simulink model "sim_pogodowa"  (R2023b)
settings: Solver=VariableStepAuto  StartTime=0.0  StopTime=10.0  FixedStep=0.1  MaxStep=10  RelTol=1e-3
model workspace (MAT data in the model file):
  Var = 0
undefined symbols (not defined in the file): ao, az, bo, bz, cpw, Cvo1, Cvo2, delta_qt1, delta_qt2, delta_Twew_SP, delta_Tzew, deltafmg1, deltafmg2, fmg1_0, fmg2_0, fmw_0, Kco, ki, kp, qt1_0, qt2_0, t_fmg1, t_fmg2, T_gp0, t_op_tr, T_oz0, t_qt1, t_qt2, t_Tzew, t_wew_SP, T_wew_SP_0, T_wp0, T_zew, T_zew0, TwzN
settings Model: Creator=tomasz  LastModifiedBy=tomasz

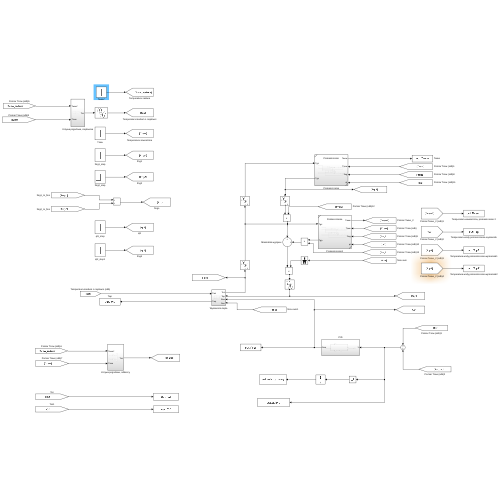
[thumbnail: Simulink's stored preview of the top-level diagram]
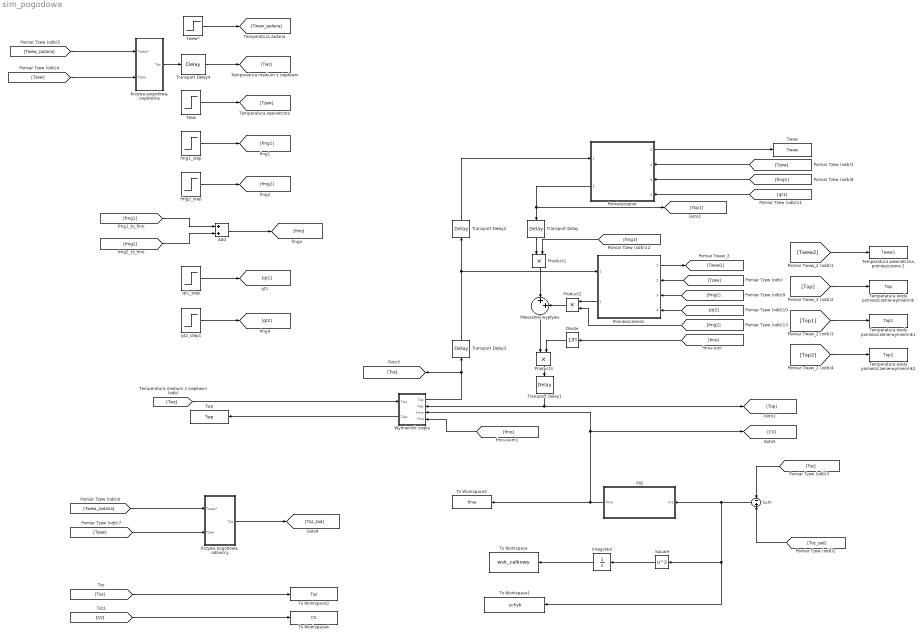
== system sim_pogodowa ==
  Add : Sum
  Divide : Product  Inputs=/
  Integrator : Integrator
  "Krzywa pogodowa, ciepłownia" : Subsystem
  "Krzywa pogodowa, odbiorcy" : Subsystem
  MIeszalnik wypływu : Sum  Inputs=|++
  PID : Subsystem
  Pomieszczenie : Subsystem  ReferencedSubsystem=Pomieszczenie
      settings: PortSchema="{\"entries\":[{\"content\":{\"sides\":[{\"content\":{\"connectorIds\":[\"In1\",\"Out1\"]},\"type\":\"ConnectorPlacement.EquallySpacedRectSide\",\"uuid\":\"8531bf00-72e2-4413-af12-728660d5b7ed\"},{\"content\":{\"connectorIds\":[\"Out2\",\"In2\",\"In3\",\"In4\"],\"side\":\"RIGHT\"},\"type\":\"ConnectorPlacement.EquallySpacedRectSide\",\"uuid\":\"61dc3c29-eecf-49ab-a3f8-5b1de1949346\"},{\"content\":{\"side\":\"TOP\"},\"type\":\"ConnectorPlacement.EquallySpacedRectSide\",\"uuid\":\"a446f5ea-277a-4598-bae9-2c6de6a131a4\"}]},\"type\":\"ConnectorPlacement.EquallySpacedConnector\",\"uuid\":\"c2b24185-542a-4b15-89a0-a367decd74d0\"}],\"packageUris\":[\"http://schema.mathworks.com/mf0/Connector/R2020b\"],\"version\":\"1.0\"}"
  Pomieszczenie1 : Subsystem  ReferencedSubsystem=Pomieszczenie
      settings: PortSchema="{\"entries\":[{\"content\":{\"sides\":[{\"content\":{\"connectorIds\":[\"In1\",\"Out1\"]},\"type\":\"ConnectorPlacement.EquallySpacedRectSide\",\"uuid\":\"8531bf00-72e2-4413-af12-728660d5b7ed\"},{\"content\":{\"connectorIds\":[\"Out2\",\"In2\",\"In3\",\"In4\"],\"side\":\"RIGHT\"},\"type\":\"ConnectorPlacement.EquallySpacedRectSide\",\"uuid\":\"61dc3c29-eecf-49ab-a3f8-5b1de1949346\"},{\"content\":{\"side\":\"TOP\"},\"type\":\"ConnectorPlacement.EquallySpacedRectSide\",\"uuid\":\"a446f5ea-277a-4598-bae9-2c6de6a131a4\"}]},\"type\":\"ConnectorPlacement.EquallySpacedConnector\",\"uuid\":\"c2b24185-542a-4b15-89a0-a367decd74d0\"}],\"packageUris\":[\"http://schema.mathworks.com/mf0/Connector/R2020b\"],\"version\":\"1.0\"}"
  Product1 : Product
  Product2 : Product
  Product3 : Product
  Square : Math  Operator=square
  Sum : Sum  Inputs=-+
  "Temperatura wewnetrzna, pomieszczenie 2" : ToWorkspace  VariableName=Twew1  SampleTime=-1
      settings: Save2DSignal=2-D array (concatenate along first dimension)
  Temperatura wody pomieszczenie-wymiennik : ToWorkspace  VariableName=Top  SampleTime=-1
      settings: Save2DSignal=2-D array (concatenate along first dimension)
  Temperatura wody pomieszczenie-wymiennik1 : ToWorkspace  VariableName=Top1  SaveFormat=Timeseries  SampleTime=-1
  Temperatura wody pomieszczenie-wymiennik2 : ToWorkspace  VariableName=Top2  SaveFormat=Timeseries  SampleTime=-1
  To Workspace : ToWorkspace  VariableName=wsk_calkowy  SampleTime=-1
  To Workspace1 : ToWorkspace  VariableName=uchyb  SampleTime=-1
  To Workspace2 : ToWorkspace  VariableName=fmw  SampleTime=-1
  To Workspace3 : ToWorkspace  VariableName=Toz  SampleTime=-1
  To Workspace4 : ToWorkspace  VariableName=CV  SampleTime=-1
      settings: Save2DSignal=2-D array (concatenate along first dimension)
  Transport Delay : TransportDelay  DelayTime=t_op_tr  InitialOutput=T_gp0
  Transport Delay1 : TransportDelay  DelayTime=t_op_tr  InitialOutput=T_gp0
  Transport Delay2 : TransportDelay  DelayTime=t_op_tr  InitialOutput=T_oz0
  Transport Delay3 : TransportDelay  DelayTime=t_op_tr  InitialOutput=T_oz0
  Transport Delay4 : TransportDelay  DelayTime=1800  InitialOutput=TwzN
  Twew : ToWorkspace  VariableName=Twew  SampleTime=-1
      settings: Save2DSignal=2-D array (concatenate along first dimension)
  Twew* : Step  Time=t_wew_SP  Before=T_wew_SP_0  After=T_wew_SP_0 + delta_Twew_SP  SampleTime=0
  Twp : ToWorkspace  VariableName=Twp  SampleTime=-1
      settings: Save2DSignal=2-D array (concatenate along first dimension)
  Tzew : Step  Time=t_Tzew  Before=T_zew0  After=T_zew + delta_Tzew  SampleTime=0
  Wymiennik ciepla : Subsystem
      settings: PortSchema="{\"entries\":[{\"content\":{\"sides\":[{\"content\":{\"connectorIds\":[\"In1\",\"Out2\"]},\"type\":\"ConnectorPlacement.EquallySpacedRectSide\",\"uuid\":\"d2a1b48e-0b7a-4274-8a7b-b9fce30bfded\"},{\"content\":{\"connectorIds\":[\"Out1\",\"In2\",\"In3\",\"In4\"],\"side\":\"RIGHT\"},\"type\":\"ConnectorPlacement.EquallySpacedRectSide\",\"uuid\":\"703c2424-3a4a-4f57-8096-11f8c1d27324\"},{\"content\":{\"side\":\"TOP\"},\"type\":\"ConnectorPlacement.EquallySpacedRectSide\",\"uuid\":\"db7a7872-15b5-4367-ab72-78f604c615eb\"},{\"content\":{\"side\":\"BOTTOM\"},\"type\":\"ConnectorPlacement.EquallySpacedRectSide\",\"uuid\":\"9424703a-0ac4-48eb-878e-9dc2ecf23458\"}]},\"type\":\"ConnectorPlacement.EquallySpacedConnector\",\"uuid\":\"032bd106-566a-41c1-86c2-0fd4a1bc5877\"}],\"packageUris\":[\"http://schema.mathworks.com/mf0/Connector/R2020b\"],\"version\":\"1.0\"}"
  fmg1_step : Step  Time=t_fmg1  Before=fmg1_0  After=fmg1_0 + deltafmg1  SampleTime=0
  fmg2_step : Step  Time=t_fmg2  Before=fmg2_0  After=fmg2_0 + deltafmg2  SampleTime=0
  qt1_step : Step  Time=t_qt1  Before=qt1_0  After=qt1_0 + delta_qt1  SampleTime=0
  qt2_step1 : Step  Time=t_qt2  Before=qt2_0  After=qt2_0 + delta_qt2  SampleTime=0
  wires:
  Pomieszczenie/2 -> Twew/1
  Pomieszczenie/1 -> Transport Delay/1, [Top1]
  Wymiennik ciepla/2(Twp) -> Twp/1
  Wymiennik ciepla/1(Toz) -> [Toz], Transport Delay3/1
  Transport Delay2/1 -> Pomieszczenie/1
  Pomieszczenie1/2 -> [Twew2]
  Twew*/1 -> [Twew_zadana]
  [Twew2] -> "Temperatura wewnetrzna, pomieszczenie 2"/1
  Tzew/1 -> [Tzew]
  [Tzew] -> Pomieszczenie1/2
  [Tzew] -> Pomieszczenie/2
  [Top] -> Temperatura wody pomieszczenie-wymiennik/1
  Transport Delay1/1 -> [Top], Wymiennik ciepla/2(Top)
  [Top1] -> Temperatura wody pomieszczenie-wymiennik1/1
  [Top2] -> Temperatura wody pomieszczenie-wymiennik2/1
  Sum/1 -> Square/1, To Workspace1/1, PID/1(In1)
  [Toz_zad] -> Sum/2
  [Toz] -> Sum/1
  Square/1 -> Integrator/1
  Integrator/1 -> To Workspace/1
  [Twz] -> Wymiennik ciepla/1(Twz)
  [Twew_zadana] -> "Krzywa pogodowa, ciepłownia"/1(Twew*)
  [Tzew] -> "Krzywa pogodowa, ciepłownia"/2(Tzew)
  "Krzywa pogodowa, ciepłownia"/1(Tsz) -> Transport Delay4/1
  Transport Delay4/1 -> [Twz]
  [Twew_zadana] -> "Krzywa pogodowa, odbiorcy"/1(Twew*)
  [Tzew] -> "Krzywa pogodowa, odbiorcy"/2(Tzew)
  "Krzywa pogodowa, odbiorcy"/1(Toz) -> [Toz_zad]
  [Toz] -> To Workspace3/1
  [fmg1] -> Pomieszczenie/3
  [fmg2] -> Pomieszczenie1/3
  [qt2] -> Pomieszczenie1/4
  [qt1] -> Pomieszczenie/4
  Transport Delay/1 -> Product1/1
  Product2/1 -> MIeszalnik wypływu/2
  Pomieszczenie1/1 -> Product2/1
  [fmg1] -> Product1/2
  [fmg2] -> Product2/2
  Product1/1 -> MIeszalnik wypływu/1
  fmg1_step/1 -> [fmg1]
  fmg2_step/1 -> [fmg2]
  [fmg1] -> Add/1
  [fmg2] -> Add/2
  Add/1 -> [fmo]
  [fmo] -> Divide/1
  [fmo] -> Wymiennik ciepla/4(fmo)
  qt1_step/1 -> [qt1]
  qt2_step1/1 -> [qt2]
  PID/1(fmw) -> [CV], Wymiennik ciepla/3(fmw), To Workspace2/1
  Transport Delay3/1 -> Transport Delay2/1, Pomieszczenie1/1
  Divide/1 -> Product3/2
  Product3/1 -> Transport Delay1/1
  MIeszalnik wypływu/1 -> Product3/1
  [CV] -> To Workspace4/1

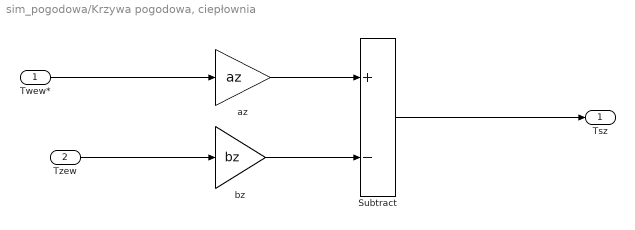
== system sim_pogodowa/Krzywa pogodowa, ciepłownia ==
  Twew* : Inport
  Tzew : Inport  Port=2
  Subtract : Sum  Inputs=+-
  az : Gain  Gain=az
  bz : Gain  Gain=bz
  Tsz : Outport
  wires:
  bz/1 -> Subtract/2
  az/1 -> Subtract/1
  Subtract/1 -> Tsz/1
  Tzew/1 -> bz/1
  Twew*/1 -> az/1

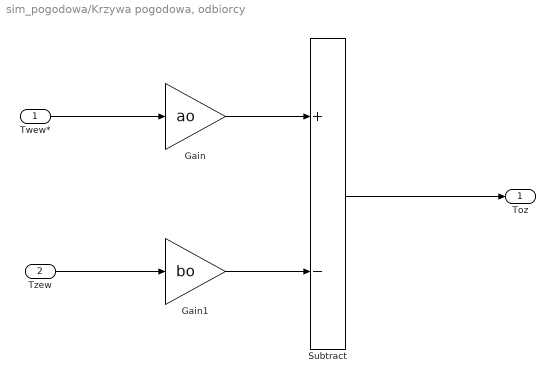
== system sim_pogodowa/Krzywa pogodowa, odbiorcy ==
  Twew* : Inport
  Tzew : Inport  Port=2
  Gain : Gain  Gain=ao
  Gain1 : Gain  Gain=bo
  Subtract : Sum  Inputs=+-
  Toz : Outport
  wires:
  Gain/1 -> Subtract/1
  Twew*/1 -> Gain/1
  Subtract/1 -> Toz/1
  Gain1/1 -> Subtract/2
  Tzew/1 -> Gain1/1

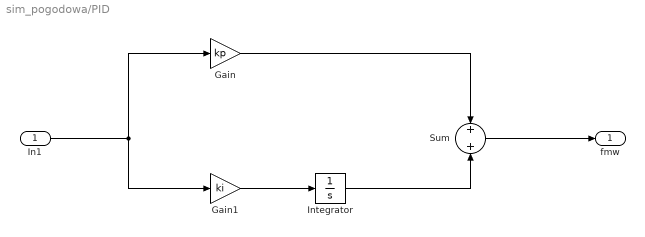
== system sim_pogodowa/PID ==
  In1 : Inport
  Gain : Gain  Gain=kp
  Gain1 : Gain  Gain=ki
  Integrator : Integrator  InitialCondition=fmw_0
  Sum : Sum
  fmw : Outport
  wires:
  Gain1/1 -> Integrator/1
  Gain/1 -> Sum/1
  In1/1 -> Gain1/1, Gain/1
  Integrator/1 -> Sum/2
  Sum/1 -> fmw/1

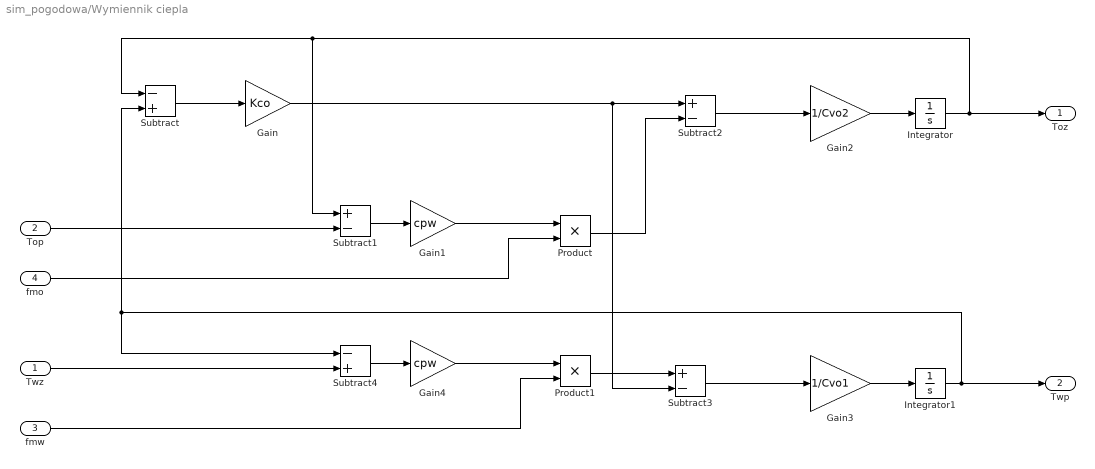
== system sim_pogodowa/Wymiennik ciepla ==
  Twz : Inport
  Top : Inport  Port=2
  fmw : Inport  Port=3
  fmo : Inport  Port=4
  Gain : Gain  Gain=Kco
  Gain1 : Gain  Gain=cpw
  Gain2 : Gain  Gain=1/Cvo2
  Gain3 : Gain  Gain=1/Cvo1
  Gain4 : Gain  Gain=cpw
  Integrator : Integrator  InitialCondition=T_oz0
  Integrator1 : Integrator  InitialCondition=T_wp0
  Product : Product
  Product1 : Product
  Subtract : Sum  Inputs=-+
  Subtract1 : Sum  Inputs=+-
  Subtract2 : Sum  Inputs=+-
  Subtract3 : Sum  Inputs=+-
  Subtract4 : Sum  Inputs=-+
  Toz : Outport
  Twp : Outport  Port=2
  wires:
  Gain4/1 -> Product1/1
  Gain3/1 -> Integrator1/1
  fmw/1 -> Product1/2
  Product/1 -> Subtract2/2
  Product1/1 -> Subtract3/1
  Integrator1/1 -> Twp/1, Subtract/2, Subtract4/1
  Gain2/1 -> Integrator/1
  Subtract4/1 -> Gain4/1
  Gain/1 -> Subtract3/2, Subtract2/1
  Top/1 -> Subtract1/2
  Subtract3/1 -> Gain3/1
  Subtract/1 -> Gain/1
  Gain1/1 -> Product/1
  Twz/1 -> Subtract4/2
  Subtract2/1 -> Gain2/1
  Subtract1/1 -> Gain1/1
  fmo/1 -> Product/2
  Integrator/1 -> Toz/1, Subtract1/1, Subtract/1
